simulink subsystem "Disturbance"  (R2024b)
settings: Solver=VariableStepAuto  StartTime=0.0  StopTime=10.0  RelTol=1e-3
undefined symbols (not defined in the file or in its folder): enable_turbulence, F, Light, MIL
libraries: aerolibwind2 x1
settings Model: Creator=thatf  LastModifiedBy=thatf

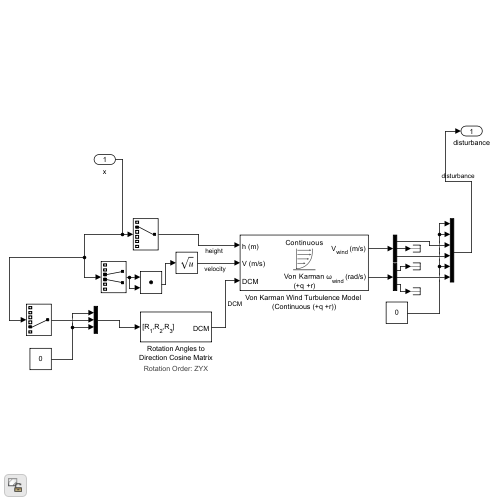
[thumbnail: Simulink's stored preview of the top-level diagram]
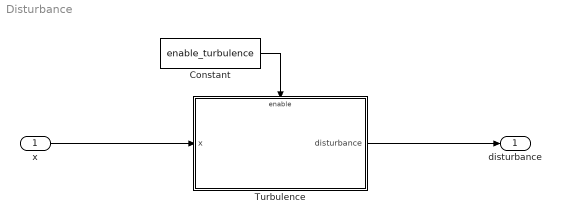
== system Disturbance ==
  x : Inport
  Constant : Constant  Value=enable_turbulence
  Turbulence : Subsystem
  disturbance : Outport
  wires:
  x/1 -> Turbulence/1(x)
  Turbulence/1(disturbance) -> disturbance/1
  Constant/1 -> Turbulence/Enable

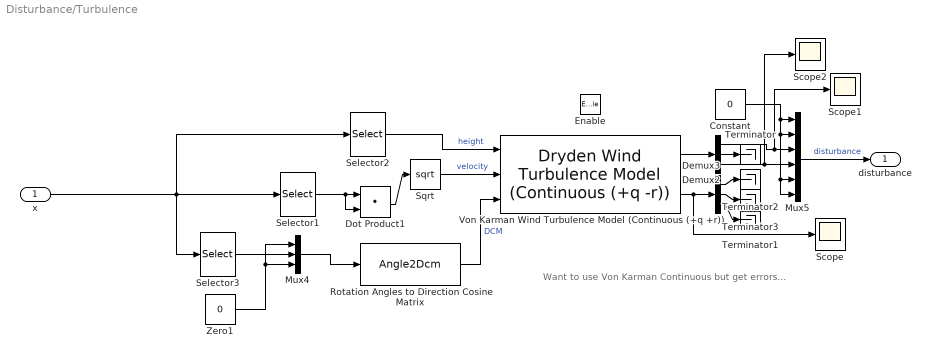
== system Disturbance/Turbulence ==
  note: Want to use Von Karman Continuous but get errors...
  x : Inport
  Enable : EnablePort
  Constant : Constant  Value=0
  Demux2 : Demux  Outputs=3
  Demux3 : Demux  Outputs=3
  Dot Product1 : DotProduct  OutDataTypeStr=Inherit: Inherit via internal rule
  Mux4 : Mux  Inputs=3
  Mux5 : Mux  Inputs=6
  Rotation Angles to Direction Cosine Matrix : Angle2Dcm
      settings: AttributesFormatString=Rotation Order: %<rotationOrder>
  Scope : Scope
  Scope1 : Scope
  Scope2 : Scope
  Selector1 : Selector  InputPortWidth=6  IndexOptions=Index vector (dialog)  Indices=[3 4]  OutputSizes=1
  Selector2 : Selector  InputPortWidth=6  IndexOptions=Index vector (dialog)  Indices=[2]  OutputSizes=1
  Selector3 : Selector  InputPortWidth=6  IndexOptions=Index vector (dialog)  Indices=[5]  OutputSizes=1
  Sqrt : Sqrt
  Terminator{,1..3} (4 alike) : Terminator
  Von Karman Wind Turbulence Model (Continuous (+q +r)) : aerolibwind2/Dryden Wind Turbulence Model  (Continuous (+q -r))  units=Metric (MKS)  spec=MIL-F-8785C  model=Discrete Dryden (+q +r)  W20=4  Wdeg=90  TurbProb=10^-2 - Light  L_high=762  Wingspan=1  ts=0.1  Seed=[23341 23342 23343 23344]  T_on=on
  Zero1 : Constant  Value=0  OutDataTypeStr=Inherit: Inherit via back propagation
  disturbance : Outport
  wires:
  Demux3/2 -> Terminator3/1
  Mux5/1 -> disturbance/1  "disturbance"
  Constant/1 -> Mux5/1, Mux5/2, Mux5/5, Mux5/6
  Rotation Angles to Direction Cosine Matrix/1 -> Von Karman Wind Turbulence Model (Continuous (+q +r))/3  "DCM"
  Demux2/3 -> Scope2/1, Mux5/4
  Selector2/1 -> Von Karman Wind Turbulence Model (Continuous (+q +r))/1  "height"
  Von Karman Wind Turbulence Model (Continuous (+q +r))/1 -> Demux2/1
  Demux2/2 -> Terminator/1
  Selector3/1 -> Mux4/2
  Selector1/1 -> Dot Product1/1, Dot Product1/2
  Von Karman Wind Turbulence Model (Continuous (+q +r))/2 -> Demux3/1, Scope/1
  x/1 -> Selector1/1, Selector3/1, Selector2/1
  Zero1/1 -> Mux4/1, Mux4/3
  Sqrt/1 -> Von Karman Wind Turbulence Model (Continuous (+q +r))/2  "velocity"
  Demux3/1 -> Terminator2/1
  Demux3/3 -> Terminator1/1
  Demux2/1 -> Mux5/3, Scope1/1
  Dot Product1/1 -> Sqrt/1
  Mux4/1 -> Rotation Angles to Direction Cosine Matrix/1
